simulink model "Step_08"  (Simulink 7.9)
settings: Solver=ode23  StartTime=0.0  StopTime=500  MaxStep=1  RelTol=1e-3
PostLoadFcn:
  | m = 150;
libraries: simulink x2, drag_library_masked x1
settings Model: Creator=wcampbel  LastModifiedBy=wcampbel
settings DebuggingCC: FcnCallInpInsideContextMsg=Use local settings  StrictBusMsg=Warning
settings GRTTargetCC: CombineOutputUpdateFcns=off  GRTInterface=on

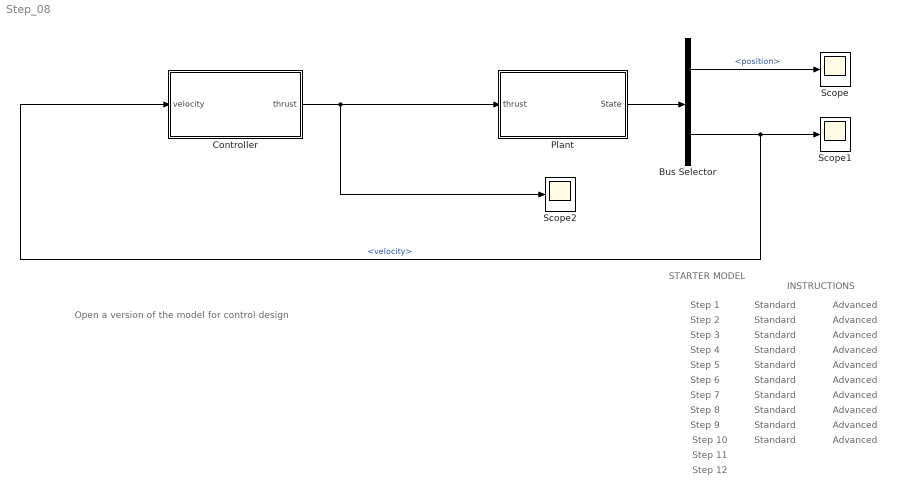
== system Step_08 ==
  note: Open a version of the model for control design
  note: Step 1
  note: Step 2
  note: Step 3
  note: STARTER
      | MODEL
  note: INSTRUCTIONS
  note: Step 4
  note: Step 5
  note: Step 6
  note: Standard
  note: Advanced
  note: Standard
  note: Advanced
  note: Standard
  note: Advanced
  note: Standard
  note: Standard
  note: Advanced
  note: Standard
  note: Advanced
  note: Step 7
  note: Step 8
  note: Step 9
  note: Step 10
  note: Step 11
  note: Standard
  note: Advanced
  note: Advanced
  note: Advanced
  note: Advanced
  note: Standard
  note: Standard
  note: Standard
  note: Advanced
  note: Step 12
  Bus Selector : BusSelector  OutputSignals=position,velocity
  Controller : Subsystem  TreatAsAtomicUnit=on
  Plant : Subsystem
  Scope : Scope
      settings: ShowLegends=on  TimeRange=500  YMin=-100  YMax=600
  Scope1 : Scope
      settings: ShowLegends=on  TimeRange=500  YMin=-25  YMax=10
  Scope2 : Scope
      settings: ShowLegends=on  TimeRange=124.5247148288973  YMin=-492.1875  YMax=1914.0625  SaveName=ScopeData2
  wires:
  Bus Selector/1 -> Scope/1  "<position>"
  Plant/1(State) -> Bus Selector/1
  Controller/1(thrust) -> Scope2/1, Plant/1(thrust)
  Bus Selector/2 -> Scope1/1, Controller/1(velocity)  "<velocity>"

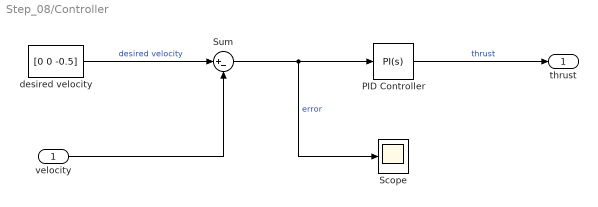
== system Step_08/Controller ==
  velocity : Inport
  PID Controller : simulink/Continuous/PID Controller  Controller=PI  TimeDomain=Continuous-time  SampleTime=1  IntegratorMethod=Forward Euler  FilterMethod=Forward Euler  Form=Parallel  P=50  I=5  D=0  N=100  InitialConditionSource=internal  InitialConditionForIntegrator=0  InitialConditionForFilter=0  ExternalReset=none  LimitOutput=off  UpperSaturationLimit=inf  LowerSaturationLimit=-inf  LinearizeAsGain=off  AntiWindupMode=none  Kb=1  TrackingMode=off  Kt=1  PParamMin=[]  PParamMax=[]  IParamMin=[]  IParamMax=[]  DParamMin=[]  DParamMax=[]  NParamMin=[]  NParamMax=[]  KbParamMin=[]  KbParamMax=[]  KtParamMin=[]  KtParamMax=[]  POutMin=[]  POutMax=[]  IOutMin=[]  IOutMax=[]  DOutMin=[]  DOutMax=[]  NOutMin=[]  NOutMax=[]  KbOutMin=[]  KbOutMax=[]  KtOutMin=[]  KtOutMax=[]  IntegratorOutMin=[]  IntegratorOutMax=[]  FilterOutMin=[]  FilterOutMax=[]  SumOutMin=[]  SumOutMax=[]  SumI1OutMin=[]  SumI1OutMax=[]  SumI2OutMin=[]  SumI2OutMax=[]  SumI3OutMin=[]  SumI3OutMax=[]  SumDOutMin=[]  SumDOutMax=[]  SaturationOutMin=[]  SaturationOutMax=[]  IntegratorContinuousStateAttributes=''  IntegratorStateMustResolveToSignalObject=off  IntegratorRTWStateStorageClass=Auto  FilterContinuousStateAttributes=''  FilterStateMustResolveToSignalObject=off  FilterRTWStateStorageClass=Auto
  Scope : Scope
      settings: TimeRange=27.56653992395438  YMin=-10  YMax=19.90625  SaveName=ScopeData3
  Sum : Sum  Inputs=|+-
  desired velocity : Constant  Value=[0 0 -0.5]
  thrust : Outport
  wires:
  desired velocity/1 -> Sum/1  "desired velocity"
  Sum/1 -> PID Controller/1, Scope/1  "error"
  velocity/1 -> Sum/2
  PID Controller/1 -> thrust/1  "thrust"

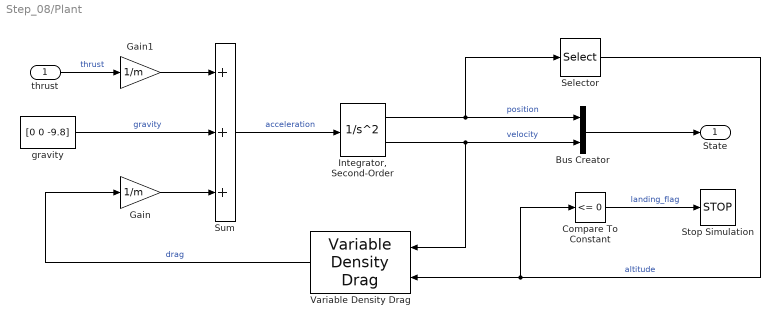
== system Step_08/Plant ==
  thrust : Inport
  Bus Creator : BusCreator  Inputs=2
  Compare To Constant : simulink/Logic and Bit Operations/Compare To Constant  relop=<=  const=0  OutDataTypeStr=boolean
  Gain : Gain  Gain=1/m
  Gain1 : Gain  Gain=1/m
  "Integrator, Second-Order" : SecondOrderIntegrator  ICX=[0 0 500]  ICDXDT=[8 -10 5]
  Selector : Selector  InputPortWidth=3  IndexOptions=Index vector (dialog)  Indices=3  OutputSizes=1
  Stop Simulation : Stop
  Sum : Sum  Inputs=+++
  Variable Density Drag : drag_library_masked/Variable Density Drag  Cd=0.333  A=1.5
  gravity : Constant  Value=[0 0 -9.8]
  State : Outport
  wires:
  "Integrator, Second-Order"/2 -> Variable Density Drag/1, Bus Creator/2  "velocity"
  Variable Density Drag/1 -> Gain/1  "drag"
  Sum/1 -> "Integrator, Second-Order"/1  "acceleration"
  thrust/1 -> Gain1/1  "thrust"
  Gain1/1 -> Sum/1
  gravity/1 -> Sum/2  "gravity"
  Gain/1 -> Sum/3
  Bus Creator/1 -> State/1
  "Integrator, Second-Order"/1 -> Bus Creator/1, Selector/1  "position"
  Selector/1 -> Variable Density Drag/2, Compare To Constant/1  "altitude"
  Compare To Constant/1 -> Stop Simulation/1  "landing_flag"
